simulink model "Exam_sim"  (R2024a)
settings: Solver=ode5  StartTime=0.0  StopTime=50  FixedStep=0.01  RelTol=1e-3
settings Model: Creator=javie  LastModifiedBy=javie

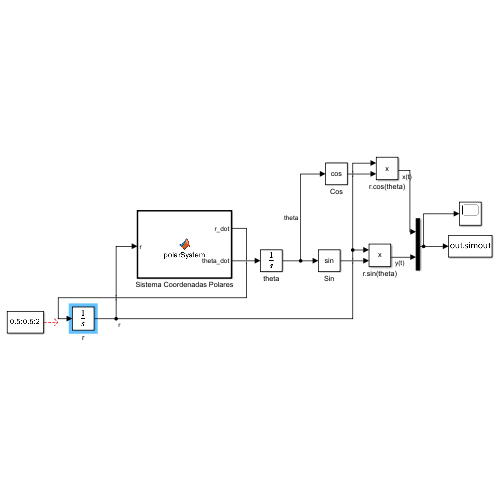
[thumbnail: Simulink's stored preview of the top-level diagram]
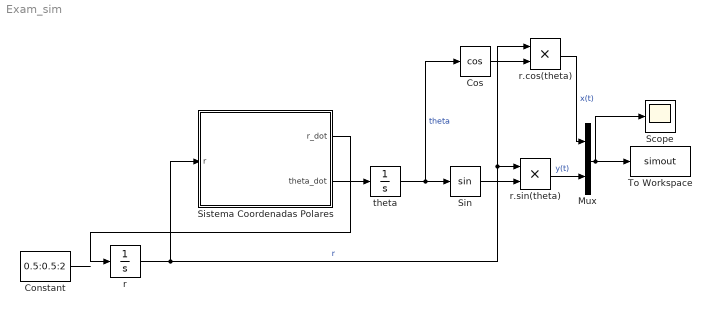
== system Exam_sim ==
  Constant : Constant  Value=0.5:0.5:2
  Cos : Trigonometry  Operator=cos
  Mux : Mux  Inputs=2
  Scope : Scope
  Sin : Trigonometry
  Sistema Coordenadas Polares : MATLAB Function  TreatAsAtomicUnit=on
  To Workspace : ToWorkspace  VariableName=simout  SaveFormat=Timeseries  SampleTime=-1
  r : Integrator  InitialCondition=0.5
  r.cos(theta) : Product
  r.sin(theta) : Product
  theta : Integrator  InitialCondition=pi/6
  wires:
  Sistema Coordenadas Polares/2(theta_dot) -> theta/1
  Constant/1 -> ?
  r/1 -> r.cos(theta)/1, r.sin(theta)/1, Sistema Coordenadas Polares/1(r)  "r"
  theta/1 -> Cos/1, Sin/1  "theta"
  Sistema Coordenadas Polares/1(r_dot) -> r/1
  Cos/1 -> r.cos(theta)/2
  Sin/1 -> r.sin(theta)/2
  r.cos(theta)/1 -> Mux/1  "x(t)"
  r.sin(theta)/1 -> Mux/2  "y(t)"
  Mux/1 -> Scope/1, To Workspace/1

== matlab function Exam_sim/Sistema Coordenadas Polares ==
  data: r input; r_dot output; theta_dot output
function [r_dot, theta_dot] = polarSystem(r)
r_dot = r.*(r-1).*(r-2);
theta_dot = pi;
end
